simulink model "gm_uz_JL_SigmaDelta_Interface"  (R2025a)
settings: Solver=FixedStepDiscrete  StartTime=0.0  StopTime=0.02  FixedStep=1e-08  RelTol=1e-3
undefined symbols (not defined in the file or in its folder): DiscIntNeverNeededParam
libraries: hdlstreaminglib x18, simulink x4, hdlsllib x2, simulink_extras x1
(part 1 of 2)
settings Model: SimulationMode=accelerator  Creator=jonat  LastModifiedBy=jonat
settings SolverCC: AlgebraicLoopSolver=TrustRegion
settings DataIOCC: LimitDataPoints=on  SaveOutput=off  SaveTime=off
settings OptimizationCC: BlockReduction=off  ConditionallyExecuteInputs=off  DefaultParameterBehavior=Inlined  InheritOutputTypeSmallerThanSingle=on  DefaultUnderspecifiedDataType=single  LifeSpan=inf
settings DebuggingCC: AlgebraicLoopMsg=error  InheritedTsInSrcMsg=none  SingleTaskRateTransMsg=error  UnconnectedInputMsg=warning  UnconnectedOutputMsg=warning  UnconnectedLineMsg=warning  AllowSymbolicDim=off  StrictBusMsg=ErrorOnBusTreatedAsVector  SFUnexpectedBacktrackingDiag=warning  SFNoUnconditionalDefaultTransitionDiag=warning  SFExecutionAtInitializationDiag=none  ArithmeticOperatorsInVariantConditions=warning
settings HardwareCC: ProdBitPerPointer=32.0  ProdBitPerSizeT=32.0  ProdBitPerPtrDiffT=32.0  ProdLargestAtomicFloat=None  ProdIntDivRoundTo=Undefined  ProdEndianess=Unspecified  ProdWordSize=32.0  ProdHWDeviceType=ASIC/FPGA->ASIC/FPGA  ProdEqTarget=off
settings ModelReferenceCC: EnableRefExpFcnMdlSchedulingChecks=on
settings SFSimCC: SimUseLocalCustomCode=off  CustomCodeUndefinedFunction=UseInterfaceOnly
settings RTWCC: RTWUseLocalCustomCode=off  GPUComputeCapability=3.5
settings CodeAppCC: StateflowObjectComments=on
settings GRTTargetCC: TargetLangStandard=C89/C90 (ANSI)
settings ConfigComp: CovScope=ReferencedModels  CovMetricSettings=dw  CovSaveCumulativeToWorkspaceVar=on  CovSaveSingleToWorkspaceVar=on  CovExternalEMLEnable=off  CovSFcnEnable=off

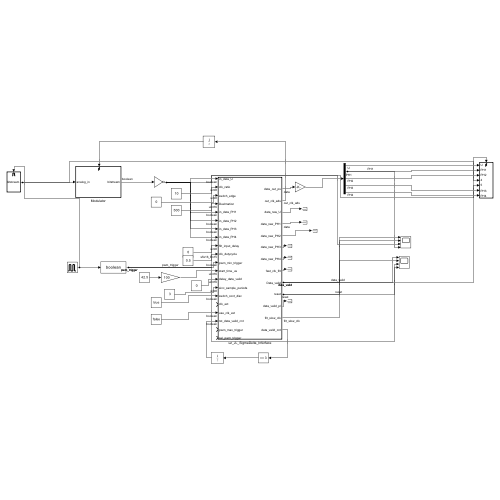
[thumbnail: Simulink's stored preview of the top-level diagram]
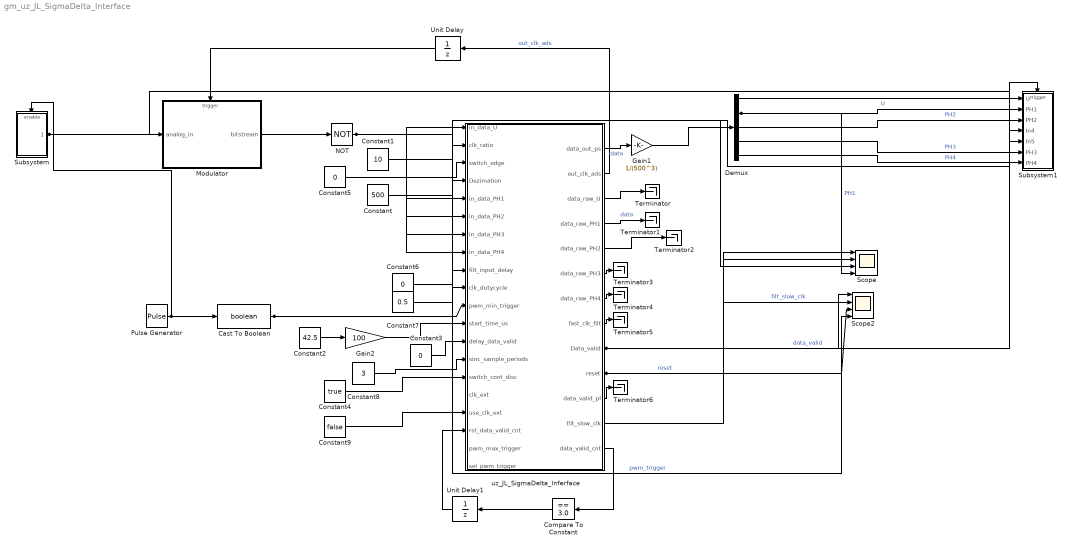
== system gm_uz_JL_SigmaDelta_Interface ==
  Cast To Boolean : DataTypeConversion  OutDataTypeStr=boolean  SaturateOnIntegerOverflow=off  RndMeth=Floor
  Compare To Constant : simulink/Logic and Bit Operations/Compare To Constant  relop===  const=3.0  OutDataTypeStr=boolean
  Constant : Constant  Value=500  OutDataTypeStr=uint16  SampleTime=-1
  Constant1 : Constant  Value=10  OutDataTypeStr=uint8  SampleTime=-1
  Constant2 : Constant  Value=42.5  OutDataTypeStr=fixdt(1,16)  SampleTime=-1
  Constant3 : Constant  Value=0  OutDataTypeStr=uint16  SampleTime=-1
  Constant4 : Constant  Value=true  OutDataTypeStr=boolean  SampleTime=-1
  Constant5 : Constant  Value=0  OutDataTypeStr=uint8  SampleTime=-1
  Constant6 : Constant  Value=0  OutDataTypeStr=uint8  SampleTime=-1
  Constant7 : Constant  Value=0.5  OutDataTypeStr=fixdt(1,16)  SampleTime=-1
  Constant8 : Constant  Value=3  OutDataTypeStr=uint8  SampleTime=-1
  Constant9 : Constant  Value=false  OutDataTypeStr=boolean  SampleTime=-1
  Demux : Demux  Outputs=5
  Gain1 : Gain  Gain=1/(500^3)
  Gain2 : Gain  Gain=100  OutDataTypeStr=uint16
  Modulator : Subsystem
  NOT : Logic  Operator=NOT  IconShape=distinctive  AllPortsSameDT=off  OutDataTypeStr=boolean
  Pulse Generator : DiscretePulseGenerator  PulseType=Time based  Period=1/10e3  PulseWidth=0.1
  Scope : Scope  NumInputPorts=4
      settings: ActiveDisplayYMinimum=-0.05268033504191956  ActiveDisplayYMaximum=1.2605943100198076
  Scope2 : Scope  NumInputPorts=4
      settings: ActiveDisplayYMinimum=-0.13880640935483335  ActiveDisplayYMaximum=1.1176045992956558  DataLoggingVariableName=ScopeData2
  Subsystem : Subsystem
  Subsystem1 : Subsystem
  Terminator{,1..6} (7 alike) : Terminator
  Unit Delay : UnitDelay  SampleTime=-1  HasFrameUpgradeWarning=on
  Unit Delay1 : UnitDelay  SampleTime=-1  HasFrameUpgradeWarning=on
  uz_JL_SigmaDelta_Inferface : Subsystem  TreatAsAtomicUnit=on
  wires:
  Demux/5 -> Subsystem1/7(PH4)  "PH4"
  Demux/4 -> Subsystem1/6(PH3)  "PH3"
  Demux/3 -> Subsystem1/3(PH2)  "PH2"
  Demux/1 -> Subsystem1/1(U)  "U"
  Subsystem/1(bitstream) -> Modulator/1(analog_in), Subsystem1/4(In4)
  Constant9/1 -> uz_JL_SigmaDelta_Inferface/17(use_clk_ext)
  Unit Delay1/1 -> uz_JL_SigmaDelta_Inferface/18(rst_data_valid_cnt)
  Compare To Constant/1 -> Unit Delay1/1
  uz_JL_SigmaDelta_Inferface/13(data_valid_cnt) -> Compare To Constant/1
  uz_JL_SigmaDelta_Inferface/12(filt_slow_clk) -> Scope2/2  "filt_slow_clk"
  NOT/1 -> uz_JL_SigmaDelta_Inferface/5(in_data_PH1), uz_JL_SigmaDelta_Inferface/6(in_data_PH2), uz_JL_SigmaDelta_Inferface/7(in_data_PH3), uz_JL_SigmaDelta_Inferface/8(in_data_PH4), uz_JL_SigmaDelta_Inferface/1(in_data_U), Subsystem1/5(In5)
  Constant4/1 -> uz_JL_SigmaDelta_Inferface/15(switch_cont_disc)
  uz_JL_SigmaDelta_Inferface/11(data_valid_pl) -> Terminator6/1
  Gain2/1 -> uz_JL_SigmaDelta_Inferface/12(start_time_us)
  Constant8/1 -> uz_JL_SigmaDelta_Inferface/14(sinc_sample_periods)
  uz_JL_SigmaDelta_Inferface/8(fast_clk_filt) -> Terminator5/1
  Gain1/1 -> Demux/1
  uz_JL_SigmaDelta_Inferface/4(data_raw_PH1) -> Terminator1/1  "data"
  Constant3/1 -> uz_JL_SigmaDelta_Inferface/13(delay_data_valid)
  uz_JL_SigmaDelta_Inferface/10(reset) -> Scope2/3, Scope/2  "reset"
  uz_JL_SigmaDelta_Inferface/9(Data_valid) -> Scope2/1, Scope/1, Subsystem1/Trigger  "data_valid"
  Cast To Boolean/1 -> uz_JL_SigmaDelta_Inferface/11(pwm_min_trigger), Scope/3, Scope2/4  "pwm_trigger"
  Pulse Generator/1 -> Cast To Boolean/1, Subsystem/Enable
  Constant2/1 -> Gain2/1
  Demux/2 -> Scope/4, Subsystem1/2(PH1)  "PH1"
  Unit Delay/1 -> Modulator/Trigger
  Modulator/1(bitstream) -> NOT/1
  uz_JL_SigmaDelta_Inferface/2(out_clk_ads) -> Unit Delay/1  "out_clk_ads"
  uz_JL_SigmaDelta_Inferface/7(data_raw_PH4) -> Terminator4/1
  uz_JL_SigmaDelta_Inferface/6(data_raw_PH3) -> Terminator3/1
  uz_JL_SigmaDelta_Inferface/5(data_raw_PH2) -> Terminator2/1
  uz_JL_SigmaDelta_Inferface/3(data_raw_U) -> Terminator/1
  uz_JL_SigmaDelta_Inferface/1(data_out_ps) -> Gain1/1  "data"
  Constant7/1 -> uz_JL_SigmaDelta_Inferface/10(clk_dutycycle)
  Constant6/1 -> uz_JL_SigmaDelta_Inferface/9(filt_input_delay)
  Constant5/1 -> uz_JL_SigmaDelta_Inferface/3(switch_edge)
  Constant1/1 -> uz_JL_SigmaDelta_Inferface/2(clk_ratio)
  Constant/1 -> uz_JL_SigmaDelta_Inferface/4(Dezimation)

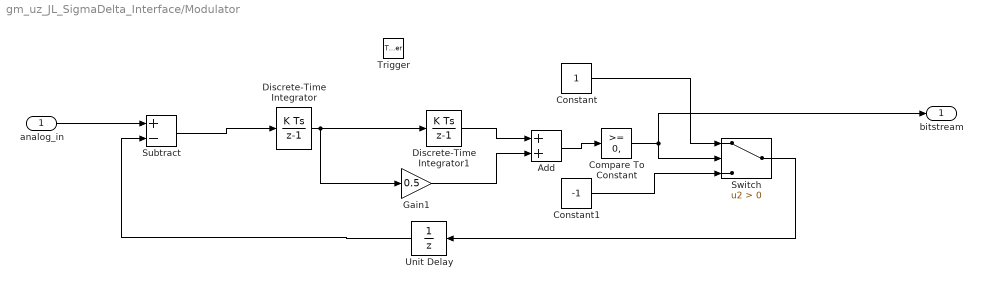
== system gm_uz_JL_SigmaDelta_Interface/Modulator ==
  analog_in : Inport
  Trigger : TriggerPort  VariantControl=(inherit)  PortDimensions=1
  Add : Sum
  Compare To Constant : simulink/Logic and Bit Operations/Compare To Constant  relop=>=  const=0,  OutDataTypeStr=boolean
  Constant : Constant
  Constant1 : Constant  Value=-1
  Discrete-Time Integrator : DiscreteIntegrator  SampleTime=-1  UpperSaturationLimit=2  LowerSaturationLimit=-2  ICPrevOutput=DiscIntNeverNeededParam  ICPrevScaledInput=DiscIntNeverNeededParam
  Discrete-Time Integrator1 : DiscreteIntegrator  SampleTime=-1  UpperSaturationLimit=2  LowerSaturationLimit=-2  ICPrevOutput=DiscIntNeverNeededParam  ICPrevScaledInput=DiscIntNeverNeededParam
  Gain1 : Gain  Gain=0.5
  Subtract : Sum  Inputs=+-  OutDataTypeStr=double
  Switch : Switch  Criteria=u2 > Threshold  OutDataTypeStr=fixdt(1,2,0)  SaturateOnIntegerOverflow=off  InputSameDT=off
  Unit Delay : UnitDelay  SampleTime=-1  HasFrameUpgradeWarning=on
  bitstream : Outport  OutDataTypeStr=boolean
  wires:
  Add/1 -> Compare To Constant/1
  Gain1/1 -> Add/2
  Unit Delay/1 -> Subtract/2
  Constant1/1 -> Switch/3
  Constant/1 -> Switch/1
  Compare To Constant/1 -> Switch/2, bitstream/1
  Switch/1 -> Unit Delay/1
  Subtract/1 -> Discrete-Time Integrator/1
  Discrete-Time Integrator1/1 -> Add/1
  Discrete-Time Integrator/1 -> Discrete-Time Integrator1/1, Gain1/1
  analog_in/1 -> Subtract/1

== system gm_uz_JL_SigmaDelta_Interface/Subsystem ==
  Enable : EnablePort
  Sine Wave : Sin  Amplitude=0.1  Frequency=2*pi*50
  bitstream : Outport
  wires:
  Sine Wave/1 -> bitstream/1  "bitstream"

== system gm_uz_JL_SigmaDelta_Interface/Subsystem1 ==
  U : Inport
  PH1 : Inport  Port=2
  PH2 : Inport  Port=3
  In4 : Inport  Port=4
  In5 : Inport  Port=5
  PH3 : Inport  Port=6
  PH4 : Inport  Port=7
  Trigger : TriggerPort  VariantControl=(inherit)  PortDimensions=1
  Scope1 : Scope  NumInputPorts=7
      settings: ActiveDisplayYMinimum=-0.12538000001752536  ActiveDisplayYMaximum=0.12538000001752536
  wires:
  U/1 -> Scope1/1
  PH3/1 -> Scope1/4
  PH1/1 -> Scope1/2
  In4/1 -> Scope1/6
  PH2/1 -> Scope1/3
  In5/1 -> Scope1/7
  PH4/1 -> Scope1/5

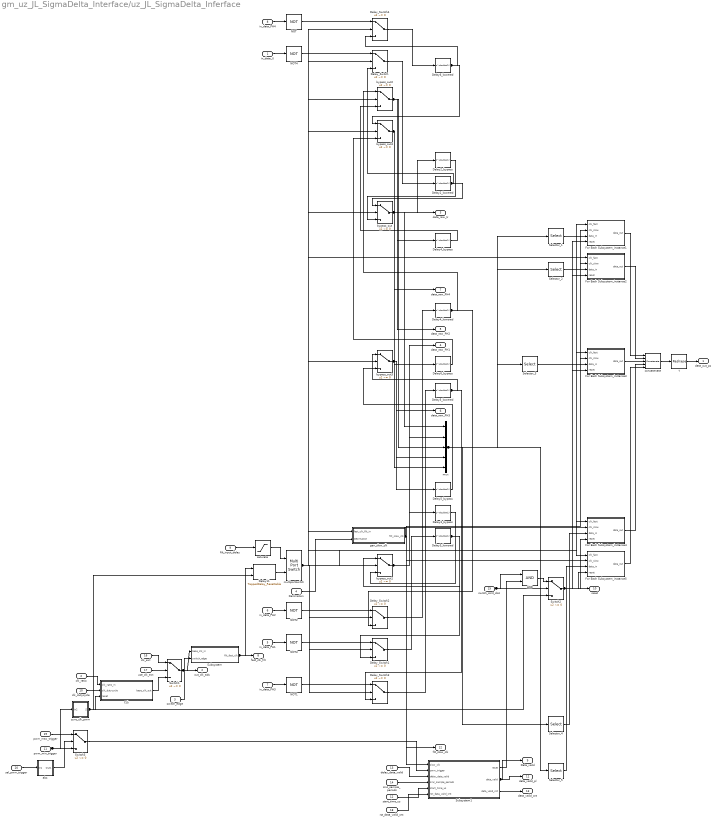
== system gm_uz_JL_SigmaDelta_Interface/uz_JL_SigmaDelta_Inferface ==
  in_data_U : Inport  OutDataTypeStr=boolean  PortDimensions=1  SampleTime=1e-08
  clk_ratio : Inport  Port=2  OutDataTypeStr=uint8  PortDimensions=1  SampleTime=1e-08
  switch_edge : Inport  Port=3  OutDataTypeStr=uint8  PortDimensions=1  SampleTime=1e-08
  Dezimation : Inport  Port=4  OutDataTypeStr=uint16  PortDimensions=1  SampleTime=1e-08
  in_data_PH1 : Inport  Port=5  OutDataTypeStr=boolean  PortDimensions=1  SampleTime=1e-08
  in_data_PH2 : Inport  Port=6  OutDataTypeStr=boolean  PortDimensions=1  SampleTime=1e-08
  in_data_PH3 : Inport  Port=7  OutDataTypeStr=boolean  PortDimensions=1  SampleTime=1e-08
  in_data_PH4 : Inport  Port=8  OutDataTypeStr=boolean  PortDimensions=1  SampleTime=1e-08
  filt_input_delay : Inport  Port=9  OutDataTypeStr=uint8  PortDimensions=1  SampleTime=1e-08
  clk_dutycycle : Inport  Port=10  OutDataTypeStr=fixdt(1, 16, 15)  PortDimensions=1  SampleTime=1e-08
  pwm_min_trigger : Inport  Port=11  OutDataTypeStr=boolean  PortDimensions=1  SampleTime=1e-08
  start_time_us : Inport  Port=12  OutDataTypeStr=uint16  PortDimensions=1  SampleTime=1e-08
  delay_data_valid : Inport  Port=13  OutDataTypeStr=uint16  PortDimensions=1  SampleTime=1e-08
  sinc_sample_periods : Inport  Port=14  OutDataTypeStr=uint8  PortDimensions=1  SampleTime=1e-08
  switch_cont_disc : Inport  Port=15  OutDataTypeStr=boolean  PortDimensions=1  SampleTime=1e-08
  clk_ext : Inport  Port=16  OutDataTypeStr=boolean  PortDimensions=1  SampleTime=1e-08
  use_clk_ext : Inport  Port=17  OutDataTypeStr=boolean  PortDimensions=1  SampleTime=1e-08
  rst_data_valid_cnt : Inport  Port=18  OutDataTypeStr=boolean  PortDimensions=1  SampleTime=1e-08
  pwm_max_trigger : Inport  Port=19  OutDataTypeStr=boolean  PortDimensions=1  SampleTime=1e-08
  sel_pwm_trigger : Inport  Port=20  OutDataTypeStr=single  PortDimensions=1  SampleTime=1e-08
  AND : Logic  AllPortsSameDT=off  OutDataTypeStr=boolean  SampleTime=1e-08
  CLk : Subsystem
  Delay11 : hdlstreaminglib/TappedDelay_Resettable  NumDelays=100  ResetTriggerType=level  DelayOrder=Newest  includeCurrent=on  samptime=-1  vinit=0
  Delay2_bypass : Delay  DelayLength=double(1)  InitialCondition=0  SampleTime=1e-08
  Delay2_lowered : Delay  DelayLength=double(1)  InitialCondition=0  SampleTime=1e-08
  Delay3_bypass : Delay  DelayLength=double(1)  InitialCondition=0  SampleTime=1e-08
  Delay3_lowered : Delay  DelayLength=double(1)  InitialCondition=0  SampleTime=1e-08
  Delay4_bypass : Delay  DelayLength=double(1)  InitialCondition=0  SampleTime=1e-08
  Delay4_lowered : Delay  DelayLength=double(1)  InitialCondition=0  SampleTime=1e-08
  Delay5_bypass : Delay  DelayLength=double(1)  InitialCondition=0  SampleTime=1e-08
  Delay5_lowered : Delay  DelayLength=double(1)  InitialCondition=0  SampleTime=1e-08
  Delay6_bypass : Delay  DelayLength=double(1)  InitialCondition=0  SampleTime=1e-08
  Delay6_lowered : Delay  DelayLength=double(1)  InitialCondition=0  SampleTime=1e-08
  Delay_Switch{,1..4} (5 alike) : Switch  Criteria=u2 ~= 0  Threshold=double(0)  OutDataTypeStr=boolean  SampleTime=1e-08  SaturateOnIntegerOverflow=off  InputSameDT=off
  For Each Subsystem_instance1 : Subsystem
  For Each Subsystem_instance2 : Subsystem
  For Each Subsystem_instance3 : Subsystem
  For Each Subsystem_instance4 : Subsystem
  For Each Subsystem_instance5 : Subsystem
  NOT{,1..4} (5 alike) : Logic  Operator=NOT  Inputs=1  AllPortsSameDT=off  OutDataTypeStr=boolean  SampleTime=1e-08
  Selector_1 : Selector  InputPortWidth=5  IndexOptions=Index vector (dialog)  Indices=double(1)  OutputSizes=1
  Selector_2 : Selector  InputPortWidth=5  IndexOptions=Index vector (dialog)  Indices=double(2)  OutputSizes=1
  Selector_3 : Selector  InputPortWidth=5  IndexOptions=Index vector (dialog)  Indices=double(3)  OutputSizes=1
  Selector_4 : Selector  InputPortWidth=5  IndexOptions=Index vector (dialog)  Indices=double(4)  OutputSizes=1
  Selector_5 : Selector  InputPortWidth=5  IndexOptions=Index vector (dialog)  Indices=double(5)  OutputSizes=1
  Subsystem : Subsystem
  Subsystem1 : Subsystem
  Switch1 : Switch  Criteria=u2 ~= 0  Threshold="fi(0,0,1,0,\"hex\",\"0\")"  OutDataTypeStr=boolean  SampleTime=1e-08  SaturateOnIntegerOverflow=off  InputSameDT=off
  Switch2 : Switch  Criteria=u2 ~= 0  Threshold="fi(0,0,1,0,\"hex\",\"0\")"  OutDataTypeStr=boolean  SampleTime=1e-08  SaturateOnIntegerOverflow=off  InputSameDT=off
  Switch3 : Switch  Criteria=u2 ~= 0  Threshold=single(0)  OutDataTypeStr=boolean  SampleTime=1e-08  SaturateOnIntegerOverflow=off  InputSameDT=off
  abs : Subsystem
      mask Display: disp('NFP\nabs');
  bypass_out{,1..4} (5 alike) : Switch  Criteria=u2 ~= 0  Threshold=double(0)  OutDataTypeStr=boolean  SampleTime=1e-08  SaturateOnIntegerOverflow=off  InputSameDT=off
  concatenate : Concatenate  NumInputs=5
  gen_slow_clk : Subsystem
  multiportswitch : MultiPortSwitch  DataPortOrder=Zero-based contiguous  Inputs=1  DiagnosticForDefault=None  zeroidx=on  SampleTime=1e-08  SaturateOnIntegerOverflow=off  InputSameDT=off
  mux : Mux  Inputs=5
  saturate : Saturate  UpperLimit=double(100)  LowerLimit=double(0)  SampleTime=1e-08  OutDataTypeStr=uint8
  sync_clk_pwm : Subsystem
  t : Reshape
  data_out_ps : Outport  SampleTime=1e-08
  out_clk_ads : Outport  Port=2  SampleTime=1e-08
  data_raw_U : Outport  Port=3  SampleTime=1e-08
  data_raw_PH1 : Outport  Port=4  SampleTime=1e-08
  data_raw_PH2 : Outport  Port=5  SampleTime=1e-08
  data_raw_PH3 : Outport  Port=6  SampleTime=1e-08
  data_raw_PH4 : Outport  Port=7  SampleTime=1e-08
  fast_clk_filt : Outport  Port=8  SampleTime=1e-08
  Data_valid : Outport  Port=9  SampleTime=1e-08
  reset : Outport  Port=10  SampleTime=1e-08
  data_valid_pl : Outport  Port=11  SampleTime=1e-08
  filt_slow_clk : Outport  Port=12  SampleTime=1e-08
  data_valid_cnt : Outport  Port=13  SampleTime=1e-08
  wires:
  sel_pwm_trigger/1 -> abs/1(In1)
  sync_clk_pwm/1(S) -> Switch2/3, Delay11/2, CLk/3(reset)
  pwm_min_trigger/1 -> Switch3/3, sync_clk_pwm/1(In2)
  switch_edge/1 -> Subsystem/2(switch_edge)
  pwm_max_trigger/1 -> Switch3/1
  abs/1(Out1) -> Switch3/2
  Delay6_lowered/1 -> bypass_out4/1, Delay_Switch4/3
  clk_dutycycle/1 -> CLk/2(clk_dutycycle)
  Selector_2/1 -> For Each Subsystem_instance2/3(data_in)
  clk_ratio/1 -> CLk/1(clk_ratio_in)
  switch_cont_disc/1 -> AND/1, Switch2/2
  Switch3/1 -> Subsystem1/2(pwm_trigger)
  clk_ext/1 -> Switch1/1
  use_clk_ext/1 -> Switch1/2
  CLk/1(base_clk_out) -> Switch1/3
  Switch1/1 -> Subsystem/1(base_clk_in), out_clk_ads/1
  Subsystem/1(filt_fast_clk) -> Delay11/1, fast_clk_filt/1
  filt_input_delay/1 -> saturate/1
  Selector_1/1 -> For Each Subsystem_instance1/3(data_in)
  in_data_PH4/1 -> NOT/1
  bypass_out/1 -> mux/1, Delay2_bypass/1, data_raw_U/1
  in_data_U/1 -> NOT4/1
  start_time_us/1 -> Subsystem1/5(start_time_us)
  saturate/1 -> multiportswitch/1
  in_data_PH1/1 -> NOT3/1
  Delay11/1 -> multiportswitch/2
  Delay6_bypass/1 -> bypass_out4/3
  in_data_PH2/1 -> NOT2/1
  in_data_PH3/1 -> NOT1/1
  sinc_sample_periods/1 -> Subsystem1/4(sinc_sample_periods)
  NOT/1 -> Delay_Switch4/1
  Dezimation/1 -> gen_slow_clk/2(Decimation)
  NOT4/1 -> Delay_Switch/1
  multiportswitch/1 -> For Each Subsystem_instance5/1(clk_fast), For Each Subsystem_instance3/1(clk_fast), For Each Subsystem_instance1/1(clk_fast), For Each Subsystem_instance4/1(clk_fast), For Each Subsystem_instance2/1(clk_fast), bypass_out4/2, Delay_Switch4/2, bypass_out3/2, bypass_out2/2, Delay_Switch2/2, bypass_out1/2, Delay_Switch1/2, bypass_out/2, Delay_Switch3/2, Delay_Switch/2, gen_slow_clk/1(fast_clk_filt_in)
  NOT2/1 -> Delay_Switch2/1
  NOT3/1 -> Delay_Switch1/1
  NOT1/1 -> Delay_Switch3/1
  gen_slow_clk/1(filt_slow_clk) -> For Each Subsystem_instance4/2(clk_slow), For Each Subsystem_instance3/2(clk_slow), For Each Subsystem_instance2/2(clk_slow), For Each Subsystem_instance5/2(clk_slow), For Each Subsystem_instance1/2(clk_slow), filt_slow_clk/1, Subsystem1/1(slow_clk)
  Selector_3/1 -> For Each Subsystem_instance3/3(data_in)
  Delay_Switch4/1 -> Delay6_lowered/1
  delay_data_valid/1 -> Subsystem1/3(delay_data_valid)
  Delay_Switch/1 -> Delay2_lowered/1
  bypass_out2/1 -> mux/3, data_raw_PH2/1, Delay4_bypass/1
  bypass_out4/1 -> Delay6_bypass/1, data_raw_PH4/1, mux/5
  bypass_out3/1 -> mux/4, Delay5_bypass/1, data_raw_PH3/1
  bypass_out1/1 -> mux/2, Delay3_bypass/1, data_raw_PH1/1
  Delay_Switch2/1 -> Delay4_lowered/1
  Delay_Switch1/1 -> Delay3_lowered/1
  Delay_Switch3/1 -> Delay5_lowered/1
  Delay4_lowered/1 -> bypass_out2/1, Delay_Switch2/3
  rst_data_valid_cnt/1 -> Subsystem1/6(rst_data_valid_cnt)
  Subsystem1/3(data_valid_cnt) -> data_valid_cnt/1
  Delay2_bypass/1 -> bypass_out/3
  Delay2_lowered/1 -> bypass_out/1, Delay_Switch/3
  Delay4_bypass/1 -> bypass_out2/3
  Delay5_lowered/1 -> bypass_out3/1, Delay_Switch3/3
  mux/1 -> Selector_5/1, Selector_4/1, Selector_2/1, Selector_1/1, Selector_3/1
  Delay5_bypass/1 -> bypass_out3/3
  Delay3_bypass/1 -> bypass_out1/3
  Delay3_lowered/1 -> Delay_Switch1/3, bypass_out1/1
  Subsystem1/1(reset) -> AND/2
  Subsystem1/2(data_valid) -> data_valid_pl/1, Data_valid/1
  AND/1 -> Switch2/1
  Switch2/1 -> For Each Subsystem_instance5/4(reset), For Each Subsystem_instance4/4(reset), For Each Subsystem_instance3/4(reset), For Each Subsystem_instance2/4(reset), For Each Subsystem_instance1/4(reset), reset/1
  Selector_4/1 -> For Each Subsystem_instance4/3(data_in)
  Selector_5/1 -> For Each Subsystem_instance5/3(data_in)
  For Each Subsystem_instance1/1(data_out) -> concatenate/1
  For Each Subsystem_instance2/1(data_out) -> concatenate/2
  For Each Subsystem_instance3/1(data_out) -> concatenate/3
  For Each Subsystem_instance4/1(data_out) -> concatenate/4
  For Each Subsystem_instance5/1(data_out) -> concatenate/5
  concatenate/1 -> t/1
  t/1 -> data_out_ps/1

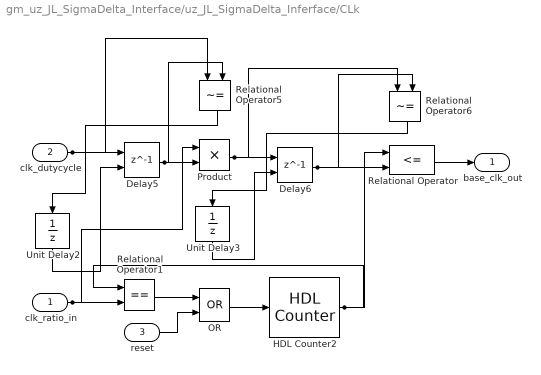
== system gm_uz_JL_SigmaDelta_Interface/uz_JL_SigmaDelta_Inferface/CLk ==
  clk_ratio_in : Inport  OutDataTypeStr=uint8  PortDimensions=1  SampleTime=1e-08
  clk_dutycycle : Inport  Port=2  OutDataTypeStr=fixdt(1, 16, 15)  PortDimensions=1  SampleTime=1e-08
  reset : Inport  Port=3  OutDataTypeStr=boolean  PortDimensions=1  SampleTime=1e-08
  Delay5 : Delay  DelayLength=1  InitialCondition=0.5  ShowEnablePort=on
      settings: InputPortMap=u0,e6
  Delay6 : Delay  DelayLength=1  InitialCondition=1  ShowEnablePort=on
      settings: InputPortMap=u0,e6
  HDL Counter2 : hdlsllib/Sources/HDL Counter  CountType=Free running  CountInit=1  CountStep=1  CountMax=25  CountFromType=Initial value  CountFrom=1  CountResetPort=on  CountLoadPort=off  CountEnbPort=off  CountDirPort=off  CountHitOutputPort=off  CountDataType=Unsigned  CountWordLen=16  CountFracLen=0  CountSampTime=1
  OR : Logic  Operator=OR  AllPortsSameDT=off  OutDataTypeStr=boolean
  Product : Product  OutMin=[1]  OutDataTypeStr=fixdt(1, 24, 15)
  Relational Operator : RelationalOperator  Operator=<=  OutDataTypeStr=boolean  RndMeth=Simplest  InputSameDT=off
  Relational Operator1 : RelationalOperator  Operator===  OutDataTypeStr=boolean  RndMeth=Simplest  InputSameDT=off
  Relational Operator5 : RelationalOperator  Operator=~=  OutDataTypeStr=boolean  RndMeth=Simplest  InputSameDT=off
  Relational Operator6 : RelationalOperator  Operator=~=  OutDataTypeStr=boolean  RndMeth=Simplest  InputSameDT=off
  Unit Delay2 : UnitDelay  InitialCondition=1  SampleTime=-1  HasFrameUpgradeWarning=on
  Unit Delay3 : UnitDelay  InitialCondition=1  SampleTime=-1  HasFrameUpgradeWarning=on
  base_clk_out : Outport  SampleTime=1e-08
  wires:
  Unit Delay2/1 -> Delay5/2
  clk_dutycycle/1 -> Relational Operator5/1, Delay5/1
  clk_ratio_in/1 -> Product/1, Relational Operator1/2
  reset/1 -> OR/2
  Product/1 -> Relational Operator6/1, Delay6/1
  Relational Operator1/1 -> OR/1
  Delay5/1 -> Relational Operator5/2, Product/2
  Relational Operator5/1 -> Unit Delay2/1
  Unit Delay3/1 -> Delay6/2
  Relational Operator6/1 -> Unit Delay3/1
  OR/1 -> HDL Counter2/1
  Delay6/1 -> Relational Operator6/2, Relational Operator/2
  HDL Counter2/1 -> Relational Operator1/1, Relational Operator/1
  Relational Operator/1 -> base_clk_out/1

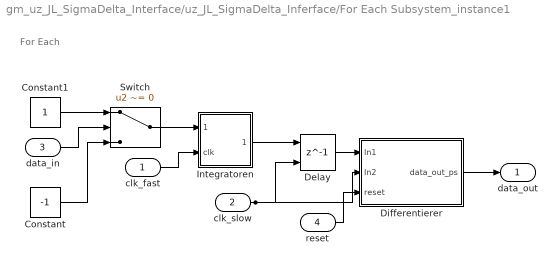
== system gm_uz_JL_SigmaDelta_Interface/uz_JL_SigmaDelta_Inferface/For Each Subsystem_instance1 ==
  note: For Each
  clk_fast : Inport  OutDataTypeStr=boolean  PortDimensions=1  SampleTime=1e-08
  clk_slow : Inport  Port=2  OutDataTypeStr=boolean  PortDimensions=1  SampleTime=1e-08
  data_in : Inport  Port=3  OutDataTypeStr=boolean  PortDimensions=1  SampleTime=1e-08
  reset : Inport  Port=4  OutDataTypeStr=boolean  PortDimensions=1  SampleTime=1e-08
  Constant : Constant  Value=-1  OutDataTypeStr=int32  SampleTime=-1
  Constant1 : Constant  OutDataTypeStr=int32  SampleTime=-1
  Delay : Delay  DelayLength=1  ShowEnablePort=on
      settings: InputPortMap=u0,e6
  Differentierer : Subsystem
  Integratoren : Subsystem
  Switch : Switch  Criteria=u2 ~= 0  OutDataTypeStr=int32  SaturateOnIntegerOverflow=off  InputSameDT=off
  data_out : Outport  SampleTime=1e-08
  wires:
  Constant1/1 -> Switch/1
  data_in/1 -> Switch/2
  Constant/1 -> Switch/3
  Switch/1 -> Integratoren/1(data)
  clk_fast/1 -> Integratoren/2(clk)
  Integratoren/1(Out1) -> Delay/1
  Delay/1 -> Differentierer/1(In1)
  clk_slow/1 -> Differentierer/2(In2), Delay/2
  reset/1 -> Differentierer/3(reset)
  Differentierer/1(data_out_ps) -> data_out/1

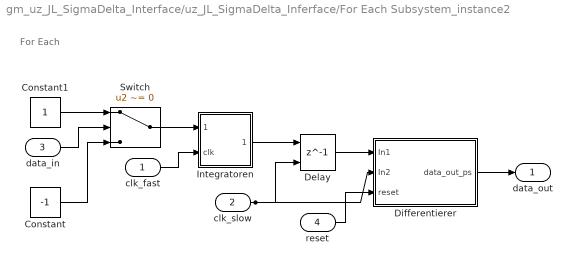
== system gm_uz_JL_SigmaDelta_Interface/uz_JL_SigmaDelta_Inferface/For Each Subsystem_instance2 ==
  note: For Each
  clk_fast : Inport  OutDataTypeStr=boolean  PortDimensions=1  SampleTime=1e-08
  clk_slow : Inport  Port=2  OutDataTypeStr=boolean  PortDimensions=1  SampleTime=1e-08
  data_in : Inport  Port=3  OutDataTypeStr=boolean  PortDimensions=1  SampleTime=1e-08
  reset : Inport  Port=4  OutDataTypeStr=boolean  PortDimensions=1  SampleTime=1e-08
  Constant : Constant  Value=-1  OutDataTypeStr=int32  SampleTime=-1
  Constant1 : Constant  OutDataTypeStr=int32  SampleTime=-1
  Delay : Delay  DelayLength=1  ShowEnablePort=on
      settings: InputPortMap=u0,e6
  Differentierer : Subsystem
  Integratoren : Subsystem
  Switch : Switch  Criteria=u2 ~= 0  OutDataTypeStr=int32  SaturateOnIntegerOverflow=off  InputSameDT=off
  data_out : Outport  SampleTime=1e-08
  wires:
  clk_slow/1 -> Differentierer/2(In2), Delay/2
  Constant1/1 -> Switch/1
  Integratoren/1(Out1) -> Delay/1
  Switch/1 -> Integratoren/1(data)
  data_in/1 -> Switch/2
  clk_fast/1 -> Integratoren/2(clk)
  Constant/1 -> Switch/3
  Delay/1 -> Differentierer/1(In1)
  reset/1 -> Differentierer/3(reset)
  Differentierer/1(data_out_ps) -> data_out/1

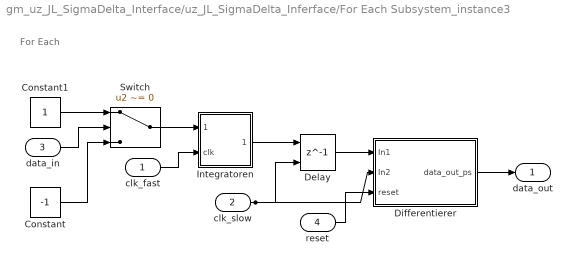
== system gm_uz_JL_SigmaDelta_Interface/uz_JL_SigmaDelta_Inferface/For Each Subsystem_instance3 ==
  note: For Each
  clk_fast : Inport  OutDataTypeStr=boolean  PortDimensions=1  SampleTime=1e-08
  clk_slow : Inport  Port=2  OutDataTypeStr=boolean  PortDimensions=1  SampleTime=1e-08
  data_in : Inport  Port=3  OutDataTypeStr=boolean  PortDimensions=1  SampleTime=1e-08
  reset : Inport  Port=4  OutDataTypeStr=boolean  PortDimensions=1  SampleTime=1e-08
  Constant : Constant  Value=-1  OutDataTypeStr=int32  SampleTime=-1
  Constant1 : Constant  OutDataTypeStr=int32  SampleTime=-1
  Delay : Delay  DelayLength=1  ShowEnablePort=on
      settings: InputPortMap=u0,e6
  Differentierer : Subsystem
  Integratoren : Subsystem
  Switch : Switch  Criteria=u2 ~= 0  OutDataTypeStr=int32  SaturateOnIntegerOverflow=off  InputSameDT=off
  data_out : Outport  SampleTime=1e-08
  wires:
  data_in/1 -> Switch/2
  Constant1/1 -> Switch/1
  Constant/1 -> Switch/3
  Switch/1 -> Integratoren/1(data)
  Delay/1 -> Differentierer/1(In1)
  clk_fast/1 -> Integratoren/2(clk)
  Integratoren/1(Out1) -> Delay/1
  clk_slow/1 -> Delay/2, Differentierer/2(In2)
  reset/1 -> Differentierer/3(reset)
  Differentierer/1(data_out_ps) -> data_out/1

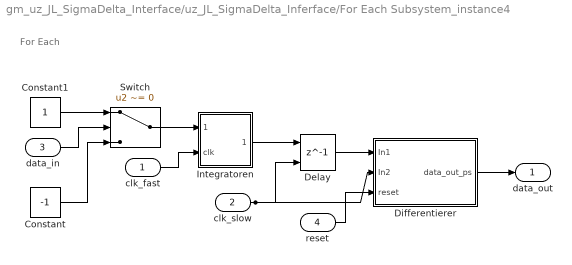
== system gm_uz_JL_SigmaDelta_Interface/uz_JL_SigmaDelta_Inferface/For Each Subsystem_instance4 ==
  note: For Each
  clk_fast : Inport  OutDataTypeStr=boolean  PortDimensions=1  SampleTime=1e-08
  clk_slow : Inport  Port=2  OutDataTypeStr=boolean  PortDimensions=1  SampleTime=1e-08
  data_in : Inport  Port=3  OutDataTypeStr=boolean  PortDimensions=1  SampleTime=1e-08
  reset : Inport  Port=4  OutDataTypeStr=boolean  PortDimensions=1  SampleTime=1e-08
  Constant : Constant  Value=-1  OutDataTypeStr=int32  SampleTime=-1
  Constant1 : Constant  OutDataTypeStr=int32  SampleTime=-1
  Delay : Delay  DelayLength=1  ShowEnablePort=on
      settings: InputPortMap=u0,e6
  Differentierer : Subsystem
  Integratoren : Subsystem
  Switch : Switch  Criteria=u2 ~= 0  OutDataTypeStr=int32  SaturateOnIntegerOverflow=off  InputSameDT=off
  data_out : Outport  SampleTime=1e-08
  wires:
  data_in/1 -> Switch/2
  Constant1/1 -> Switch/1
  Constant/1 -> Switch/3
  Switch/1 -> Integratoren/1(data)
  clk_fast/1 -> Integratoren/2(clk)
  clk_slow/1 -> Differentierer/2(In2), Delay/2
  Integratoren/1(Out1) -> Delay/1
  Delay/1 -> Differentierer/1(In1)
  reset/1 -> Differentierer/3(reset)
  Differentierer/1(data_out_ps) -> data_out/1

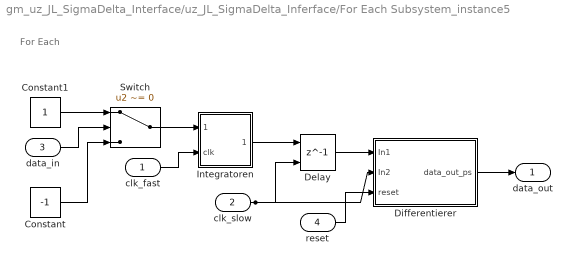
== system gm_uz_JL_SigmaDelta_Interface/uz_JL_SigmaDelta_Inferface/For Each Subsystem_instance5 ==
  note: For Each
  clk_fast : Inport  OutDataTypeStr=boolean  PortDimensions=1  SampleTime=1e-08
  clk_slow : Inport  Port=2  OutDataTypeStr=boolean  PortDimensions=1  SampleTime=1e-08
  data_in : Inport  Port=3  OutDataTypeStr=boolean  PortDimensions=1  SampleTime=1e-08
  reset : Inport  Port=4  OutDataTypeStr=boolean  PortDimensions=1  SampleTime=1e-08
  Constant : Constant  Value=-1  OutDataTypeStr=int32  SampleTime=-1
  Constant1 : Constant  OutDataTypeStr=int32  SampleTime=-1
  Delay : Delay  DelayLength=1  ShowEnablePort=on
      settings: InputPortMap=u0,e6
  Differentierer : Subsystem
  Integratoren : Subsystem
  Switch : Switch  Criteria=u2 ~= 0  OutDataTypeStr=int32  SaturateOnIntegerOverflow=off  InputSameDT=off
  data_out : Outport  SampleTime=1e-08
  wires:
  data_in/1 -> Switch/2
  Constant1/1 -> Switch/1
  Constant/1 -> Switch/3
  Switch/1 -> Integratoren/1(data)
  Delay/1 -> Differentierer/1(In1)
  clk_fast/1 -> Integratoren/2(clk)
  clk_slow/1 -> Differentierer/2(In2), Delay/2
  Integratoren/1(Out1) -> Delay/1
  reset/1 -> Differentierer/3(reset)
  Differentierer/1(data_out_ps) -> data_out/1

== system gm_uz_JL_SigmaDelta_Interface/uz_JL_SigmaDelta_Inferface/Subsystem ==
  base_clk_in : Inport  OutDataTypeStr=boolean  PortDimensions=1  SampleTime=1e-08
  switch_edge : Inport  Port=2  OutDataTypeStr=uint8  PortDimensions=1  SampleTime=1e-08
  Logical Operator : Logic  Operator=OR  AllPortsSameDT=off  OutDataTypeStr=boolean
  Switch1 : Switch  Criteria=u2 ~= 0  OutDataTypeStr=boolean  SaturateOnIntegerOverflow=off  InputSameDT=off
  Switch2 : Switch  Criteria=u2 > Threshold  Threshold=1  OutDataTypeStr=boolean  SaturateOnIntegerOverflow=off  InputSameDT=off
  trigger_sec_edge : Subsystem
  filt_fast_clk : Outport  SampleTime=1e-08
  wires:
  base_clk_in/1 -> trigger_sec_edge/1(trigger_in)
  switch_edge/1 -> Switch1/2, Switch2/2
  Switch2/1 -> Switch1/1
  trigger_sec_edge/1(trigger_1_3) -> Switch2/1, Logical Operator/1
  Switch1/1 -> filt_fast_clk/1
  trigger_sec_edge/2(trigger_2_4) -> Switch2/3, Logical Operator/2
  Logical Operator/1 -> Switch1/3

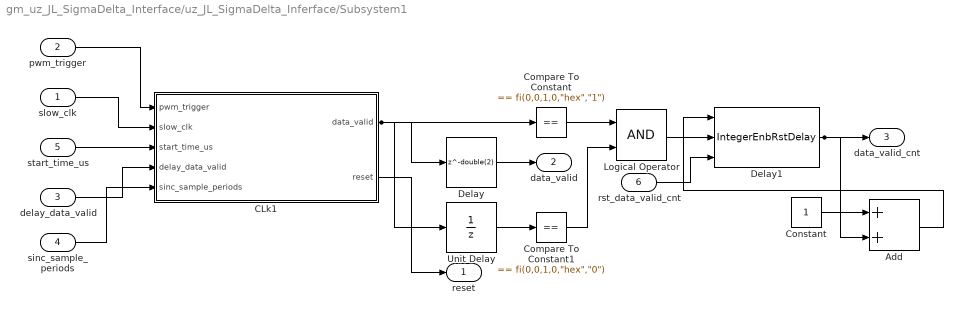
== system gm_uz_JL_SigmaDelta_Interface/uz_JL_SigmaDelta_Inferface/Subsystem1 ==
  slow_clk : Inport  OutDataTypeStr=boolean  PortDimensions=1  SampleTime=1e-08
  pwm_trigger : Inport  Port=2  OutDataTypeStr=boolean  PortDimensions=1  SampleTime=1e-08
  delay_data_valid : Inport  Port=3  OutDataTypeStr=uint16  PortDimensions=1  SampleTime=1e-08
  sinc_sample_periods : Inport  Port=4  OutDataTypeStr=uint8  PortDimensions=1  SampleTime=1e-08
  start_time_us : Inport  Port=5  OutDataTypeStr=uint16  PortDimensions=1  SampleTime=1e-08
  rst_data_valid_cnt : Inport  Port=6  OutDataTypeStr=boolean  PortDimensions=1  SampleTime=1e-08
  Add : Sum  OutDataTypeStr=uint8  AccumDataTypeStr=uint8  SampleTime=1e-08
  CLk1 : Subsystem
  Compare To Constant : simulink/Logic and Bit Operations/Compare To Constant  relop===  const="fi(0,0,1,0,\"hex\",\"1\")"  OutDataTypeStr=boolean
  Compare To Constant1 : simulink/Logic and Bit Operations/Compare To Constant  relop===  const="fi(0,0,1,0,\"hex\",\"0\")"  OutDataTypeStr=boolean
  Constant : Constant  OutDataTypeStr=uint8  SampleTime=1e-08
  Delay : Delay  DelayLength=double(2)  InitialCondition=0  SampleTime=1e-08
  Delay1 : hdlstreaminglib/IntegerEnbRstDelay  ExternalReset=Level  InitialCondition=0  DelayLength=1  StopWhenAssertionFail=on
  Logical Operator : Logic  AllPortsSameDT=off  OutDataTypeStr=boolean  SampleTime=1e-08
  Unit Delay : UnitDelay  SampleTime=1e-08
  reset : Outport  SampleTime=1e-08
  data_valid : Outport  Port=2  SampleTime=1e-08
  data_valid_cnt : Outport  Port=3  OutDataTypeStr=uint8  SampleTime=1e-08
  wires:
  Logical Operator/1 -> Delay1/2
  pwm_trigger/1 -> CLk1/1(pwm_trigger)
  slow_clk/1 -> CLk1/2(slow_clk)
  CLk1/2(reset) -> reset/1
  start_time_us/1 -> CLk1/3(start_time_us)
  delay_data_valid/1 -> CLk1/4(delay_data_valid)
  sinc_sample_periods/1 -> CLk1/5(sinc_sample_periods)
  CLk1/1(data_valid) -> Compare To Constant/1, Unit Delay/1, Delay/1
  Delay/1 -> data_valid/1
  Unit Delay/1 -> Compare To Constant1/1
  Compare To Constant/1 -> Logical Operator/1
  rst_data_valid_cnt/1 -> Delay1/3
  Compare To Constant1/1 -> Logical Operator/2
  Delay1/1 -> Add/2, data_valid_cnt/1
  Constant/1 -> Add/1
  Add/1 -> Delay1/1

== system gm_uz_JL_SigmaDelta_Interface/uz_JL_SigmaDelta_Inferface/abs ==
  In1 : Inport
  abs : Abs  SampleTime=1e-08  OutDataTypeStr=single  SaturateOnIntegerOverflow=off
  Out1 : Outport
  wires:
  In1/1 -> abs/1
  abs/1 -> Out1/1

== system gm_uz_JL_SigmaDelta_Interface/uz_JL_SigmaDelta_Inferface/gen_slow_clk ==
  fast_clk_filt_in : Inport  OutDataTypeStr=boolean  PortDimensions=1  SampleTime=1e-08
  Decimation : Inport  Port=2  OutDataTypeStr=uint16  PortDimensions=1  SampleTime=1e-08
  Add : Sum  OutDataTypeStr=fixdt(1,32,0)
  Constant : Constant  OutDataTypeStr=fixdt(1,32,0)  SampleTime=-1
  Constant1 : Constant  Value=0  OutDataTypeStr=fixdt(1,32,0)  SampleTime=-1
  Delay : Delay  DelayLength=1  InitialCondition=0  ExternalReset=Level
      settings: InputPortMap=u0,r5
  Delay1 : Delay  DelayLength=1
  Logical Operator : Logic  AllPortsSameDT=off  OutDataTypeStr=boolean
  Relational Operator : RelationalOperator  OutDataTypeStr=boolean  RndMeth=Simplest  InputSameDT=off
  Switch : Switch  Criteria=u2 ~= 0  OutDataTypeStr=fixdt(1,32,0)  SaturateOnIntegerOverflow=off  InputSameDT=off
  filt_slow_clk : Outport  SampleTime=1e-08
  wires:
  Constant1/1 -> Switch/3
  Decimation/1 -> Relational Operator/2
  Constant/1 -> Switch/1
  Switch/1 -> Add/2
  fast_clk_filt_in/1 -> Switch/2, Logical Operator/1
  Relational Operator/1 -> Delay1/1, Logical Operator/2
  Delay1/1 -> Delay/2
  Logical Operator/1 -> filt_slow_clk/1
  Delay/1 -> Add/1
  Add/1 -> Relational Operator/1, Delay/1

== system gm_uz_JL_SigmaDelta_Interface/uz_JL_SigmaDelta_Inferface/sync_clk_pwm ==
  In2 : Inport  OutDataTypeStr=boolean  PortDimensions=1  SampleTime=1e-08
  Constant : Constant  OutDataTypeStr=boolean  SampleTime=-1
  Constant1 : Constant  Value=0  OutDataTypeStr=boolean  SampleTime=-1
  Constant2 : Constant  Value=0  OutDataTypeStr=boolean  SampleTime=-1
  Logical Operator1 : Logic  AllPortsSameDT=off  OutDataTypeStr=boolean
  S-R Flip-Flop : simulink_extras/Flip Flops/S-R Flip-Flop  initial_condition=0
  S-R Flip-Flop_inst_term1 : Terminator
  Switch2 : Switch  Criteria=u2 > Threshold  OutDataTypeStr=boolean  SaturateOnIntegerOverflow=off  InputSameDT=off
  Unit Delay : UnitDelay  SampleTime=-1  HasFrameUpgradeWarning=on
  S : Outport  SampleTime=1e-08
  wires:
  In2/1 -> Logical Operator1/2
  Constant1/1 -> Switch2/1
  Constant/1 -> Switch2/3
  Unit Delay/1 -> Switch2/2
  Switch2/1 -> Logical Operator1/1
  S-R Flip-Flop/1 -> Unit Delay/1
  Logical Operator1/1 -> S/1, S-R Flip-Flop/1
  Constant2/1 -> S-R Flip-Flop/2
  S-R Flip-Flop/2 -> S-R Flip-Flop_inst_term1/1

== system gm_uz_JL_SigmaDelta_Interface/uz_JL_SigmaDelta_Inferface/For Each Subsystem_instance1/Differentierer ==
  note: Differnetiatior3
  note: Differnetiatior2
  note: Differnetiatior
  In1 : Inport  OutDataTypeStr=int32  PortDimensions=1  SampleTime=1e-08
  In2 : Inport  Port=2  OutDataTypeStr=boolean  PortDimensions=1  SampleTime=1e-08
  reset : Inport  Port=3  OutDataTypeStr=boolean  PortDimensions=1  SampleTime=1e-08
  Delay One Step1 : hdlstreaminglib/IntegerEnbRstDelay  ExternalReset=Level  InitialCondition=0  DelayLength=1  StopWhenAssertionFail=on
  Delay One Step2 : hdlstreaminglib/IntegerEnbRstDelay  ExternalReset=Level  InitialCondition=0  DelayLength=1  StopWhenAssertionFail=on
  Delay One Step3 : hdlstreaminglib/IntegerEnbRstDelay  ExternalReset=Level  InitialCondition=0  DelayLength=1  StopWhenAssertionFail=on
  Sub_Comp1 : Sum  Inputs=+-  OutDataTypeStr=int32  AccumDataTypeStr=int32  SampleTime=1e-08
  Sub_Comp2 : Sum  Inputs=+-  OutDataTypeStr=int32  AccumDataTypeStr=int32  SampleTime=1e-08
  Sub_Comp3 : Sum  Inputs=+-  OutDataTypeStr=int32  AccumDataTypeStr=int32  SampleTime=1e-08
  data_out_ps : Outport  SampleTime=1e-08
  wires:
  Delay One Step1/1 -> Sub_Comp1/2
  In1/1 -> Sub_Comp1/1, Delay One Step1/1
  In2/1 -> Delay One Step2/2, Delay One Step3/2, Delay One Step1/2
  reset/1 -> Delay One Step2/3, Delay One Step3/3, Delay One Step1/3
  Sub_Comp1/1 -> Sub_Comp2/1, Delay One Step2/1
  Delay One Step2/1 -> Sub_Comp2/2
  Delay One Step3/1 -> Sub_Comp3/2
  Sub_Comp2/1 -> Sub_Comp3/1, Delay One Step3/1
  Sub_Comp3/1 -> data_out_ps/1

== system gm_uz_JL_SigmaDelta_Interface/uz_JL_SigmaDelta_Inferface/For Each Subsystem_instance1/Integratoren ==
  note: Integrator
  note: Integrator1
  note: Integrator2
  data : Inport  OutDataTypeStr=int32  PortDimensions=1  SampleTime=1e-08
  clk : Inport  Port=2  OutDataTypeStr=boolean  PortDimensions=1  SampleTime=1e-08
  Add_Int1 : Sum  OutDataTypeStr=int32
  Add_Int2 : Sum  OutDataTypeStr=int32
  Add_Int3 : Sum  OutDataTypeStr=int32
  Delay One Step4 : Delay  DelayLength=1  ShowEnablePort=on
      settings: InputPortMap=u0,e6
  Delay One Step5 : Delay  DelayLength=1  ShowEnablePort=on
      settings: InputPortMap=u0,e6
  Delay One Step6 : Delay  DelayLength=1  ShowEnablePort=on
      settings: InputPortMap=u0,e6
  Out1 : Outport  SampleTime=1e-08
  wires:
  Delay One Step4/1 -> Add_Int1/1, Add_Int2/2
  clk/1 -> Delay One Step4/2, Delay One Step5/2, Delay One Step6/2
  Delay One Step6/1 -> Add_Int3/1, Out1/1
  data/1 -> Add_Int1/2
  Delay One Step5/1 -> Add_Int2/1, Add_Int3/2
  Add_Int3/1 -> Delay One Step6/1
  Add_Int2/1 -> Delay One Step5/1
  Add_Int1/1 -> Delay One Step4/1

== system gm_uz_JL_SigmaDelta_Interface/uz_JL_SigmaDelta_Inferface/For Each Subsystem_instance2/Differentierer ==
  note: Differnetiatior
  note: Differnetiatior2
  note: Differnetiatior3
  In1 : Inport  OutDataTypeStr=int32  PortDimensions=1  SampleTime=1e-08
  In2 : Inport  Port=2  OutDataTypeStr=boolean  PortDimensions=1  SampleTime=1e-08
  reset : Inport  Port=3  OutDataTypeStr=boolean  PortDimensions=1  SampleTime=1e-08
  Delay One Step1 : hdlstreaminglib/IntegerEnbRstDelay  ExternalReset=Level  InitialCondition=0  DelayLength=1  StopWhenAssertionFail=on
  Delay One Step2 : hdlstreaminglib/IntegerEnbRstDelay  ExternalReset=Level  InitialCondition=0  DelayLength=1  StopWhenAssertionFail=on
  Delay One Step3 : hdlstreaminglib/IntegerEnbRstDelay  ExternalReset=Level  InitialCondition=0  DelayLength=1  StopWhenAssertionFail=on
  Sub_Comp1 : Sum  Inputs=+-  OutDataTypeStr=int32  AccumDataTypeStr=int32  SampleTime=1e-08
  Sub_Comp2 : Sum  Inputs=+-  OutDataTypeStr=int32  AccumDataTypeStr=int32  SampleTime=1e-08
  Sub_Comp3 : Sum  Inputs=+-  OutDataTypeStr=int32  AccumDataTypeStr=int32  SampleTime=1e-08
  data_out_ps : Outport  SampleTime=1e-08
  wires:
  Sub_Comp3/1 -> data_out_ps/1
  Sub_Comp2/1 -> Delay One Step3/1, Sub_Comp3/1
  Delay One Step3/1 -> Sub_Comp3/2
  Delay One Step2/1 -> Sub_Comp2/2
  Sub_Comp1/1 -> Delay One Step2/1, Sub_Comp2/1
  reset/1 -> Delay One Step1/3, Delay One Step3/3, Delay One Step2/3
  In2/1 -> Delay One Step1/2, Delay One Step3/2, Delay One Step2/2
  In1/1 -> Delay One Step1/1, Sub_Comp1/1
  Delay One Step1/1 -> Sub_Comp1/2

== system gm_uz_JL_SigmaDelta_Interface/uz_JL_SigmaDelta_Inferface/For Each Subsystem_instance2/Integratoren ==
  note: Integrator2
  note: Integrator1
  note: Integrator
  data : Inport  OutDataTypeStr=int32  PortDimensions=1  SampleTime=1e-08
  clk : Inport  Port=2  OutDataTypeStr=boolean  PortDimensions=1  SampleTime=1e-08
  Add_Int1 : Sum  OutDataTypeStr=int32
  Add_Int2 : Sum  OutDataTypeStr=int32
  Add_Int3 : Sum  OutDataTypeStr=int32
  Delay One Step4 : Delay  DelayLength=1  ShowEnablePort=on
      settings: InputPortMap=u0,e6
  Delay One Step5 : Delay  DelayLength=1  ShowEnablePort=on
      settings: InputPortMap=u0,e6
  Delay One Step6 : Delay  DelayLength=1  ShowEnablePort=on
      settings: InputPortMap=u0,e6
  Out1 : Outport  SampleTime=1e-08
  wires:
  Add_Int1/1 -> Delay One Step4/1
  Add_Int2/1 -> Delay One Step5/1
  Add_Int3/1 -> Delay One Step6/1
  Delay One Step5/1 -> Add_Int3/2, Add_Int2/1
  data/1 -> Add_Int1/2
  Delay One Step6/1 -> Out1/1, Add_Int3/1
  clk/1 -> Delay One Step6/2, Delay One Step5/2, Delay One Step4/2
  Delay One Step4/1 -> Add_Int2/2, Add_Int1/1

== system gm_uz_JL_SigmaDelta_Interface/uz_JL_SigmaDelta_Inferface/For Each Subsystem_instance3/Differentierer ==
  note: Differnetiatior
  note: Differnetiatior2
  note: Differnetiatior3
  In1 : Inport  OutDataTypeStr=int32  PortDimensions=1  SampleTime=1e-08
  In2 : Inport  Port=2  OutDataTypeStr=boolean  PortDimensions=1  SampleTime=1e-08
  reset : Inport  Port=3  OutDataTypeStr=boolean  PortDimensions=1  SampleTime=1e-08
  Delay One Step1 : hdlstreaminglib/IntegerEnbRstDelay  ExternalReset=Level  InitialCondition=0  DelayLength=1  StopWhenAssertionFail=on
  Delay One Step2 : hdlstreaminglib/IntegerEnbRstDelay  ExternalReset=Level  InitialCondition=0  DelayLength=1  StopWhenAssertionFail=on
  Delay One Step3 : hdlstreaminglib/IntegerEnbRstDelay  ExternalReset=Level  InitialCondition=0  DelayLength=1  StopWhenAssertionFail=on
  Sub_Comp1 : Sum  Inputs=+-  OutDataTypeStr=int32  AccumDataTypeStr=int32  SampleTime=1e-08
  Sub_Comp2 : Sum  Inputs=+-  OutDataTypeStr=int32  AccumDataTypeStr=int32  SampleTime=1e-08
  Sub_Comp3 : Sum  Inputs=+-  OutDataTypeStr=int32  AccumDataTypeStr=int32  SampleTime=1e-08
  data_out_ps : Outport  SampleTime=1e-08
  wires:
  Sub_Comp3/1 -> data_out_ps/1
  Sub_Comp2/1 -> Delay One Step3/1, Sub_Comp3/1
  Delay One Step3/1 -> Sub_Comp3/2
  Delay One Step2/1 -> Sub_Comp2/2
  Sub_Comp1/1 -> Delay One Step2/1, Sub_Comp2/1
  reset/1 -> Delay One Step1/3, Delay One Step3/3, Delay One Step2/3
  In2/1 -> Delay One Step1/2, Delay One Step3/2, Delay One Step2/2
  In1/1 -> Delay One Step1/1, Sub_Comp1/1
  Delay One Step1/1 -> Sub_Comp1/2

== system gm_uz_JL_SigmaDelta_Interface/uz_JL_SigmaDelta_Inferface/For Each Subsystem_instance3/Integratoren ==
  note: Integrator2
  note: Integrator1
  note: Integrator
  data : Inport  OutDataTypeStr=int32  PortDimensions=1  SampleTime=1e-08
  clk : Inport  Port=2  OutDataTypeStr=boolean  PortDimensions=1  SampleTime=1e-08
  Add_Int1 : Sum  OutDataTypeStr=int32
  Add_Int2 : Sum  OutDataTypeStr=int32
  Add_Int3 : Sum  OutDataTypeStr=int32
  Delay One Step4 : Delay  DelayLength=1  ShowEnablePort=on
      settings: InputPortMap=u0,e6
  Delay One Step5 : Delay  DelayLength=1  ShowEnablePort=on
      settings: InputPortMap=u0,e6
  Delay One Step6 : Delay  DelayLength=1  ShowEnablePort=on
      settings: InputPortMap=u0,e6
  Out1 : Outport  SampleTime=1e-08
  wires:
  Add_Int1/1 -> Delay One Step4/1
  Add_Int2/1 -> Delay One Step5/1
  Add_Int3/1 -> Delay One Step6/1
  Delay One Step5/1 -> Add_Int3/2, Add_Int2/1
  data/1 -> Add_Int1/2
  Delay One Step6/1 -> Out1/1, Add_Int3/1
  clk/1 -> Delay One Step6/2, Delay One Step5/2, Delay One Step4/2
  Delay One Step4/1 -> Add_Int2/2, Add_Int1/1

== system gm_uz_JL_SigmaDelta_Interface/uz_JL_SigmaDelta_Inferface/For Each Subsystem_instance4/Differentierer ==
  note: Differnetiatior
  note: Differnetiatior2
  note: Differnetiatior3
  In1 : Inport  OutDataTypeStr=int32  PortDimensions=1  SampleTime=1e-08
  In2 : Inport  Port=2  OutDataTypeStr=boolean  PortDimensions=1  SampleTime=1e-08
  reset : Inport  Port=3  OutDataTypeStr=boolean  PortDimensions=1  SampleTime=1e-08
  Delay One Step1 : hdlstreaminglib/IntegerEnbRstDelay  ExternalReset=Level  InitialCondition=0  DelayLength=1  StopWhenAssertionFail=on
  Delay One Step2 : hdlstreaminglib/IntegerEnbRstDelay  ExternalReset=Level  InitialCondition=0  DelayLength=1  StopWhenAssertionFail=on
  Delay One Step3 : hdlstreaminglib/IntegerEnbRstDelay  ExternalReset=Level  InitialCondition=0  DelayLength=1  StopWhenAssertionFail=on
  Sub_Comp1 : Sum  Inputs=+-  OutDataTypeStr=int32  AccumDataTypeStr=int32  SampleTime=1e-08
  Sub_Comp2 : Sum  Inputs=+-  OutDataTypeStr=int32  AccumDataTypeStr=int32  SampleTime=1e-08
  Sub_Comp3 : Sum  Inputs=+-  OutDataTypeStr=int32  AccumDataTypeStr=int32  SampleTime=1e-08
  data_out_ps : Outport  SampleTime=1e-08
  wires:
  Sub_Comp3/1 -> data_out_ps/1
  Sub_Comp2/1 -> Delay One Step3/1, Sub_Comp3/1
  Delay One Step3/1 -> Sub_Comp3/2
  Delay One Step2/1 -> Sub_Comp2/2
  Sub_Comp1/1 -> Delay One Step2/1, Sub_Comp2/1
  reset/1 -> Delay One Step1/3, Delay One Step3/3, Delay One Step2/3
  In2/1 -> Delay One Step1/2, Delay One Step3/2, Delay One Step2/2
  In1/1 -> Delay One Step1/1, Sub_Comp1/1
  Delay One Step1/1 -> Sub_Comp1/2

== system gm_uz_JL_SigmaDelta_Interface/uz_JL_SigmaDelta_Inferface/For Each Subsystem_instance4/Integratoren ==
  note: Integrator2
  note: Integrator1
  note: Integrator
  data : Inport  OutDataTypeStr=int32  PortDimensions=1  SampleTime=1e-08
  clk : Inport  Port=2  OutDataTypeStr=boolean  PortDimensions=1  SampleTime=1e-08
  Add_Int1 : Sum  OutDataTypeStr=int32
  Add_Int2 : Sum  OutDataTypeStr=int32
  Add_Int3 : Sum  OutDataTypeStr=int32
  Delay One Step4 : Delay  DelayLength=1  ShowEnablePort=on
      settings: InputPortMap=u0,e6
  Delay One Step5 : Delay  DelayLength=1  ShowEnablePort=on
      settings: InputPortMap=u0,e6
  Delay One Step6 : Delay  DelayLength=1  ShowEnablePort=on
      settings: InputPortMap=u0,e6
  Out1 : Outport  SampleTime=1e-08
  wires:
  Add_Int1/1 -> Delay One Step4/1
  Add_Int2/1 -> Delay One Step5/1
  Add_Int3/1 -> Delay One Step6/1
  Delay One Step5/1 -> Add_Int3/2, Add_Int2/1
  data/1 -> Add_Int1/2
  Delay One Step6/1 -> Out1/1, Add_Int3/1
  clk/1 -> Delay One Step6/2, Delay One Step5/2, Delay One Step4/2
  Delay One Step4/1 -> Add_Int2/2, Add_Int1/1

== system gm_uz_JL_SigmaDelta_Interface/uz_JL_SigmaDelta_Inferface/For Each Subsystem_instance5/Differentierer ==
  note: Differnetiatior
  note: Differnetiatior2
  note: Differnetiatior3
  In1 : Inport  OutDataTypeStr=int32  PortDimensions=1  SampleTime=1e-08
  In2 : Inport  Port=2  OutDataTypeStr=boolean  PortDimensions=1  SampleTime=1e-08
  reset : Inport  Port=3  OutDataTypeStr=boolean  PortDimensions=1  SampleTime=1e-08
  Delay One Step1 : hdlstreaminglib/IntegerEnbRstDelay  ExternalReset=Level  InitialCondition=0  DelayLength=1  StopWhenAssertionFail=on
  Delay One Step2 : hdlstreaminglib/IntegerEnbRstDelay  ExternalReset=Level  InitialCondition=0  DelayLength=1  StopWhenAssertionFail=on
  Delay One Step3 : hdlstreaminglib/IntegerEnbRstDelay  ExternalReset=Level  InitialCondition=0  DelayLength=1  StopWhenAssertionFail=on
  Sub_Comp1 : Sum  Inputs=+-  OutDataTypeStr=int32  AccumDataTypeStr=int32  SampleTime=1e-08
  Sub_Comp2 : Sum  Inputs=+-  OutDataTypeStr=int32  AccumDataTypeStr=int32  SampleTime=1e-08
  Sub_Comp3 : Sum  Inputs=+-  OutDataTypeStr=int32  AccumDataTypeStr=int32  SampleTime=1e-08
  data_out_ps : Outport  SampleTime=1e-08
  wires:
  Sub_Comp3/1 -> data_out_ps/1
  Sub_Comp2/1 -> Delay One Step3/1, Sub_Comp3/1
  Delay One Step3/1 -> Sub_Comp3/2
  Delay One Step2/1 -> Sub_Comp2/2
  Sub_Comp1/1 -> Delay One Step2/1, Sub_Comp2/1
  reset/1 -> Delay One Step1/3, Delay One Step3/3, Delay One Step2/3
  In2/1 -> Delay One Step1/2, Delay One Step3/2, Delay One Step2/2
  In1/1 -> Delay One Step1/1, Sub_Comp1/1
  Delay One Step1/1 -> Sub_Comp1/2

== system gm_uz_JL_SigmaDelta_Interface/uz_JL_SigmaDelta_Inferface/For Each Subsystem_instance5/Integratoren ==
  note: Integrator2
  note: Integrator1
  note: Integrator
  data : Inport  OutDataTypeStr=int32  PortDimensions=1  SampleTime=1e-08
  clk : Inport  Port=2  OutDataTypeStr=boolean  PortDimensions=1  SampleTime=1e-08
  Add_Int1 : Sum  OutDataTypeStr=int32
  Add_Int2 : Sum  OutDataTypeStr=int32
  Add_Int3 : Sum  OutDataTypeStr=int32
  Delay One Step4 : Delay  DelayLength=1  ShowEnablePort=on
      settings: InputPortMap=u0,e6
  Delay One Step5 : Delay  DelayLength=1  ShowEnablePort=on
      settings: InputPortMap=u0,e6
  Delay One Step6 : Delay  DelayLength=1  ShowEnablePort=on
      settings: InputPortMap=u0,e6
  Out1 : Outport  SampleTime=1e-08
  wires:
  Add_Int1/1 -> Delay One Step4/1
  Add_Int2/1 -> Delay One Step5/1
  Add_Int3/1 -> Delay One Step6/1
  Delay One Step5/1 -> Add_Int3/2, Add_Int2/1
  data/1 -> Add_Int1/2
  Delay One Step6/1 -> Out1/1, Add_Int3/1
  clk/1 -> Delay One Step6/2, Delay One Step5/2, Delay One Step4/2
  Delay One Step4/1 -> Add_Int2/2, Add_Int1/1

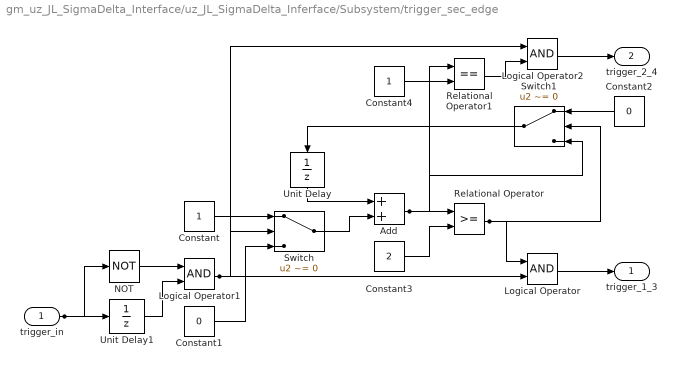
== system gm_uz_JL_SigmaDelta_Interface/uz_JL_SigmaDelta_Inferface/Subsystem/trigger_sec_edge ==
  trigger_in : Inport  OutDataTypeStr=boolean  PortDimensions=1  SampleTime=1e-08
  Add : Sum  OutDataTypeStr=fixdt(1,32,0)
  Constant : Constant  OutDataTypeStr=fixdt(1,32,0)  SampleTime=-1
  Constant1 : Constant  Value=0  OutDataTypeStr=fixdt(1,32,0)  SampleTime=-1
  Constant2 : Constant  Value=0  OutDataTypeStr=fixdt(1,32,0)  SampleTime=-1
  Constant3 : Constant  Value=2  OutDataTypeStr=fixdt(1,32,0)  SampleTime=-1
  Constant4 : Constant  OutDataTypeStr=fixdt(1,32,0)  SampleTime=-1
  Logical Operator : Logic  AllPortsSameDT=off  OutDataTypeStr=boolean
  Logical Operator1 : Logic  AllPortsSameDT=off  OutDataTypeStr=boolean
  Logical Operator2 : Logic  AllPortsSameDT=off  OutDataTypeStr=boolean
  NOT : Logic  Operator=NOT  IconShape=distinctive  AllPortsSameDT=off  OutDataTypeStr=boolean
  Relational Operator : RelationalOperator  OutDataTypeStr=boolean  RndMeth=Simplest  InputSameDT=off
  Relational Operator1 : RelationalOperator  Operator===  OutDataTypeStr=boolean  RndMeth=Simplest  InputSameDT=off
  Switch : Switch  Criteria=u2 ~= 0  OutDataTypeStr=fixdt(1,32,0)  SaturateOnIntegerOverflow=off  InputSameDT=off
  Switch1 : Switch  Criteria=u2 ~= 0  OutDataTypeStr=fixdt(1,32,0)  SaturateOnIntegerOverflow=off  InputSameDT=off
  Unit Delay : UnitDelay  SampleTime=-1  HasFrameUpgradeWarning=on
  Unit Delay1 : UnitDelay  SampleTime=-1  HasFrameUpgradeWarning=on
  trigger_1_3 : Outport  SampleTime=1e-08
  trigger_2_4 : Outport  Port=2  SampleTime=1e-08
  wires:
  trigger_in/1 -> NOT/1, Unit Delay1/1
  NOT/1 -> Logical Operator1/1
  Switch/1 -> Add/2
  Unit Delay1/1 -> Logical Operator1/2
  Constant/1 -> Switch/1
  Logical Operator1/1 -> Logical Operator2/1, Logical Operator/2, Switch/2
  Constant1/1 -> Switch/3
  Unit Delay/1 -> Add/1
  Constant4/1 -> Relational Operator1/2
  Constant2/1 -> Switch1/1
  Add/1 -> Switch1/3, Relational Operator1/1, Relational Operator/1
  Constant3/1 -> Relational Operator/2
  Relational Operator1/1 -> Logical Operator2/2
  Relational Operator/1 -> Switch1/2, Logical Operator/1
  Switch1/1 -> Unit Delay/1
  Logical Operator2/1 -> trigger_2_4/1
  Logical Operator/1 -> trigger_1_3/1
